simulink model "Tra_DblClthDet"  (R2016b)
settings: configuration reference "CodeGenConfigSet" (kept outside this file)
values from neighbouring files (symbols this model uses):
  Tra_trqDblClthEngMax_C = Calibration.Parameter    [init_Tra_DblClthDet.m]
  Tra_trqDblClthVehMax_C = Calibration.Parameter    [init_Tra_DblClthDet.m]
settings Model: Creator=Colin  LastModifiedBy=lenovo
settings ConfigSetRef: SourceLocation=Base Workspace

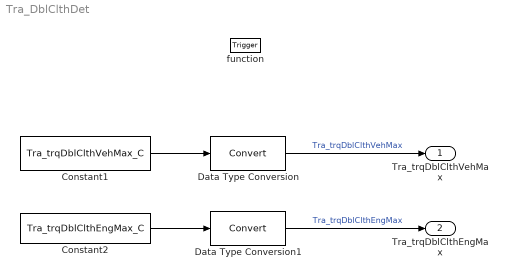
== system Tra_DblClthDet ==
  function : TriggerPort  TriggerType=function-call  VariantControl=Variant
  Constant1 : Constant  Value=Tra_trqDblClthVehMax_C  OutDataTypeStr=Trq_Nm
  Constant2 : Constant  Value=Tra_trqDblClthEngMax_C  OutDataTypeStr=Trq_Nm
  Data Type Conversion : DataTypeConversion
  Data Type Conversion1 : DataTypeConversion
  Tra_trqDblClthVehMax : Outport  Tag=Nm  Description=minimum torque of highest speed limitation Nm  OutMin=-3000  OutMax=3000  OutDataTypeStr=Trq_Nm
  Tra_trqDblClthEngMax : Outport  Tag=Nm  Description=Application parameter for minimum torque of systemdegratation Nm  Port=2  OutMin=-3000  OutMax=3000  OutDataTypeStr=Trq_Nm
  wires:
  Constant1/1 -> Data Type Conversion/1
  Constant2/1 -> Data Type Conversion1/1
  Data Type Conversion/1 -> Tra_trqDblClthVehMax/1  "Tra_trqDblClthVehMax"
  Data Type Conversion1/1 -> Tra_trqDblClthEngMax/1  "Tra_trqDblClthEngMax"
